simulink model "Copy_of_DiscreteSystem_manual_discrete_controller"  (R2024b)
settings: Solver=VariableStepAuto  StartTime=0.0  StopTime=20.0  RelTol=1e-3
values from neighbouring files (symbols this model uses):
  disorder_times = [10, 14]    [assignment1.m]
  sys_d = c2d(sys, Ts)    [assignment1.m]
  u_control = 0.5    [assignment1.m]
  z = 0.1    [assignment1.m]
undefined symbols (not defined in the file or in its folder): P, Q
settings Model: Creator=lukiq  LastModifiedBy=lukiq

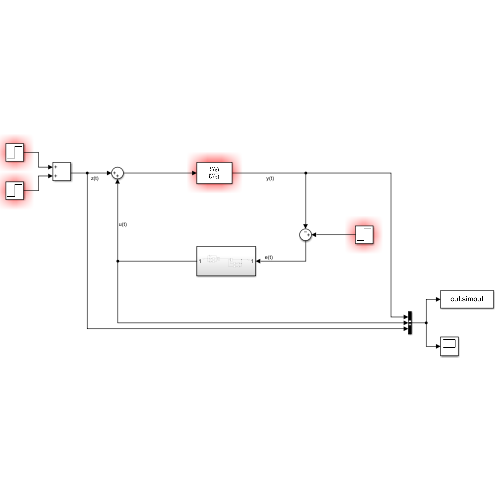
[thumbnail: Simulink's stored preview of the top-level diagram]
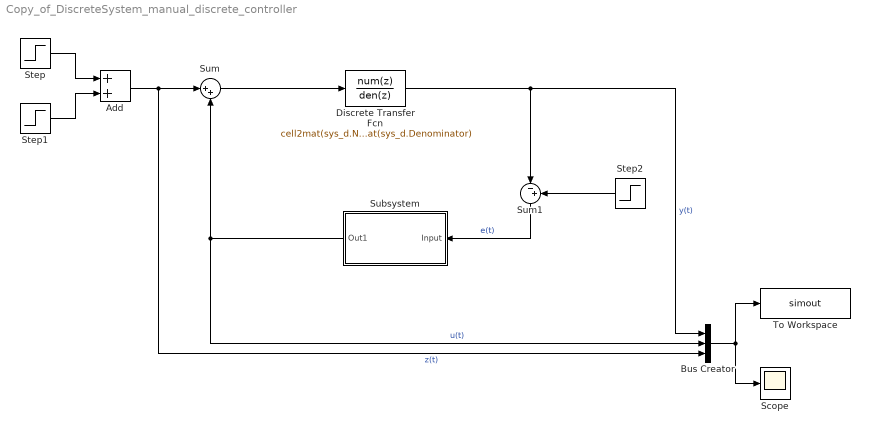
== system Copy_of_DiscreteSystem_manual_discrete_controller ==
  Add : Sum
  Bus Creator : BusCreator  Inputs=3
  Discrete Transfer Fcn : DiscreteTransferFcn  Numerator=cell2mat(sys_d.Numerator)  Denominator=cell2mat(sys_d.Denominator)
  Scope : Scope
  Step : Step  Time=disorder_times(1)  After=z * u_control  SampleTime=0
  Step1 : Step  Time=disorder_times(2)  After=-z * u_control  SampleTime=0
  Step2 : Step  Time=0  After=u_control  SampleTime=0
  Subsystem : Subsystem
  Sum : Sum  Inputs=|++
  Sum1 : Sum  Inputs=|-+
  To Workspace : ToWorkspace  VariableName=simout  SaveFormat=Timeseries  SampleTime=-1
  wires:
  Subsystem/1(Out1) -> Bus Creator/2, Sum/2  "u(t)"
  Step/1 -> Add/1
  Add/1 -> Bus Creator/3, Sum/1  "z(t)"
  Step2/1 -> Sum1/2
  Sum1/1 -> Subsystem/1(Input)  "e(t)"
  Discrete Transfer Fcn/1 -> Bus Creator/1, Sum1/1  "y(t)"
  Step1/1 -> Add/2
  Bus Creator/1 -> Scope/1, To Workspace/1
  Sum/1 -> Discrete Transfer Fcn/1

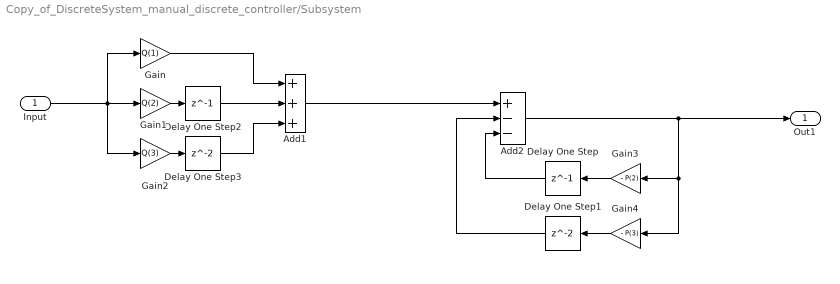
== system Copy_of_DiscreteSystem_manual_discrete_controller/Subsystem ==
  Input : Inport
  Add1 : Sum  Inputs=+++
  Add2 : Sum  Inputs=+--
  Delay One Step : Delay  DelayLength=1
  Delay One Step1 : Delay
  Delay One Step2 : Delay  DelayLength=1
  Delay One Step3 : Delay
  Gain : Gain  Gain=Q(1)
  Gain1 : Gain  Gain=Q(2)
  Gain2 : Gain  Gain=Q(3)
  Gain3 : Gain  Gain=- P(2)
  Gain4 : Gain  Gain=- P(3)
  Out1 : Outport
  wires:
  Gain2/1 -> Delay One Step3/1
  Gain/1 -> Add1/1
  Add1/1 -> Add2/1
  Add2/1 -> Out1/1, Gain3/1, Gain4/1
  Delay One Step/1 -> Add2/3
  Gain1/1 -> Delay One Step2/1
  Delay One Step1/1 -> Add2/2
  Gain3/1 -> Delay One Step/1
  Delay One Step3/1 -> Add1/3
  Input/1 -> Gain2/1, Gain1/1, Gain/1
  Gain4/1 -> Delay One Step1/1
  Delay One Step2/1 -> Add1/2
